simulink model "stormAD_Architecture"  (R2024a)
settings: Solver=FixedStepDiscrete  StartTime=0.0  StopTime=10.0  RelTol=1e-3
model workspace (MAT data in the model file):
  bstInterface : Simulink.Bus (value not decoded)
undefined symbols (not defined in the file): orig, RepoFilePath, UI, VisualizeDataset
(part 3 of 3)

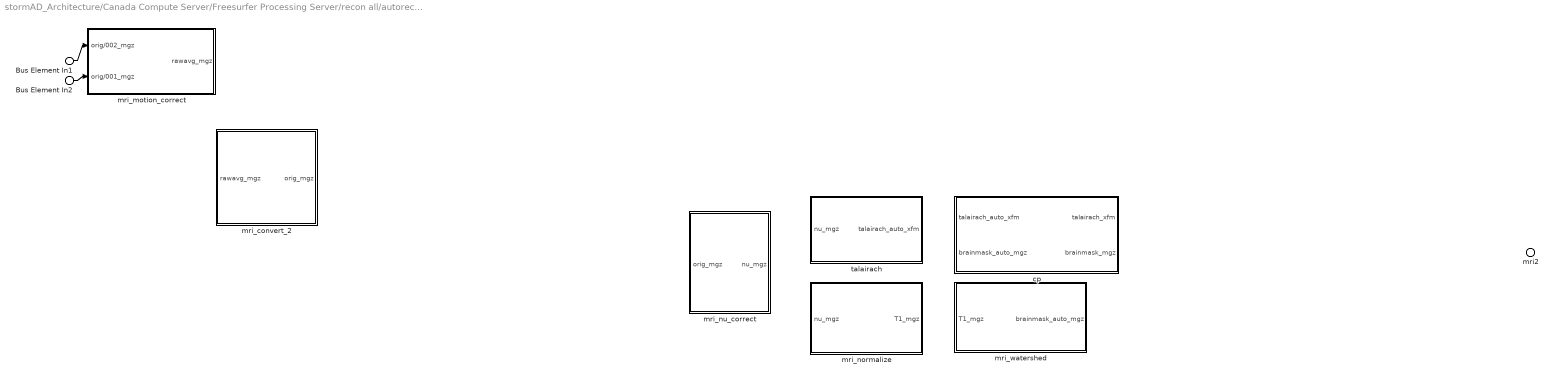
== system stormAD_Architecture/Canada Compute Server/Freesurfer Processing Server/recon all/autorecon1 ==
  Bus Element In2 : Inport  PortName=orig/001_mgz
  Bus Element In1 : Inport  Port=2  PortName=orig/002_mgz
  cp : Subsystem
      settings: PortSchema="{\"entries\":[{\"content\":{\"headerSize\":26,\"margin\":15,\"minimumSpacing\":25,\"sides\":[{\"content\":{\"connectorIds\":[\"In1\",\"In2\"]},\"type\":\"ConnectorPlacement.EquallySpacedRectSide\",\"uuid\":\"d99db108-8c8a-4010-81b2-f142fbf318f5\"},{\"content\":{\"connectorIds\":[\"Out1\",\"Out2\"],\"side\":\"RIGHT\"},\"type\":\"ConnectorPlacement.EquallySpacedRectSide\",\"uuid\":\"9190d96c-22e3-4cc9-a507-8f094dc67743\"},{\"content\":{\"side\":\"TOP\"},\"type\":\"ConnectorPlacement.EquallySpacedRectSide\",\"uuid\":\"08b46875-eac1-4edb-b2eb-5598dd517a75\"}]},\"type\":\"ConnectorPlacement.EquallySpacedConnector\",\"uuid\":\"c8d2d02b-cf5a-431f-8876-22d36c8a9b33\"}],\"packageUris\":[\"http://schema.mathworks.com/mf0/Connector/R2020b\"],\"version\":\"1.0\"}"
  mri_convert_2 : Subsystem
      settings: PortSchema="{\"entries\":[{\"content\":{\"headerSize\":26,\"margin\":15,\"minimumSpacing\":25,\"sides\":[{\"content\":{\"connectorIds\":[\"In1\"]},\"type\":\"ConnectorPlacement.EquallySpacedRectSide\",\"uuid\":\"d99db108-8c8a-4010-81b2-f142fbf318f5\"},{\"content\":{\"connectorIds\":[\"Out1\"],\"side\":\"RIGHT\"},\"type\":\"ConnectorPlacement.EquallySpacedRectSide\",\"uuid\":\"9190d96c-22e3-4cc9-a507-8f094dc67743\"},{\"content\":{\"side\":\"TOP\"},\"type\":\"ConnectorPlacement.EquallySpacedRectSide\",\"uuid\":\"08b46875-eac1-4edb-b2eb-5598dd517a75\"}]},\"type\":\"ConnectorPlacement.EquallySpacedConnector\",\"uuid\":\"c8d2d02b-cf5a-431f-8876-22d36c8a9b33\"}],\"packageUris\":[\"http://schema.mathworks.com/mf0/Connector/R2020b\"],\"version\":\"1.0\"}"
  mri_motion_correct : Subsystem
      settings: PortSchema="{\"entries\":[{\"content\":{\"headerSize\":26,\"margin\":15,\"minimumSpacing\":25,\"sides\":[{\"content\":{\"connectorIds\":[\"In1\",\"In2\"]},\"type\":\"ConnectorPlacement.EquallySpacedRectSide\",\"uuid\":\"d99db108-8c8a-4010-81b2-f142fbf318f5\"},{\"content\":{\"connectorIds\":[\"Out1\"],\"side\":\"RIGHT\"},\"type\":\"ConnectorPlacement.EquallySpacedRectSide\",\"uuid\":\"9190d96c-22e3-4cc9-a507-8f094dc67743\"},{\"content\":{\"side\":\"TOP\"},\"type\":\"ConnectorPlacement.EquallySpacedRectSide\",\"uuid\":\"08b46875-eac1-4edb-b2eb-5598dd517a75\"}]},\"type\":\"ConnectorPlacement.EquallySpacedConnector\",\"uuid\":\"c8d2d02b-cf5a-431f-8876-22d36c8a9b33\"}],\"packageUris\":[\"http://schema.mathworks.com/mf0/Connector/R2020b\"],\"version\":\"1.0\"}"
  mri_normalize : Subsystem
      settings: PortSchema="{\"entries\":[{\"content\":{\"headerSize\":26,\"margin\":15,\"minimumSpacing\":25,\"sides\":[{\"content\":{\"connectorIds\":[\"In1\"]},\"type\":\"ConnectorPlacement.EquallySpacedRectSide\",\"uuid\":\"d99db108-8c8a-4010-81b2-f142fbf318f5\"},{\"content\":{\"connectorIds\":[\"Out1\"],\"side\":\"RIGHT\"},\"type\":\"ConnectorPlacement.EquallySpacedRectSide\",\"uuid\":\"9190d96c-22e3-4cc9-a507-8f094dc67743\"},{\"content\":{\"side\":\"TOP\"},\"type\":\"ConnectorPlacement.EquallySpacedRectSide\",\"uuid\":\"08b46875-eac1-4edb-b2eb-5598dd517a75\"}]},\"type\":\"ConnectorPlacement.EquallySpacedConnector\",\"uuid\":\"c8d2d02b-cf5a-431f-8876-22d36c8a9b33\"}],\"packageUris\":[\"http://schema.mathworks.com/mf0/Connector/R2020b\"],\"version\":\"1.0\"}"
  mri_nu_correct : Subsystem
      settings: PortSchema="{\"entries\":[{\"content\":{\"headerSize\":26,\"margin\":15,\"minimumSpacing\":25,\"sides\":[{\"content\":{\"connectorIds\":[\"In1\"]},\"type\":\"ConnectorPlacement.EquallySpacedRectSide\",\"uuid\":\"d99db108-8c8a-4010-81b2-f142fbf318f5\"},{\"content\":{\"connectorIds\":[\"Out1\"],\"side\":\"RIGHT\"},\"type\":\"ConnectorPlacement.EquallySpacedRectSide\",\"uuid\":\"9190d96c-22e3-4cc9-a507-8f094dc67743\"},{\"content\":{\"side\":\"TOP\"},\"type\":\"ConnectorPlacement.EquallySpacedRectSide\",\"uuid\":\"08b46875-eac1-4edb-b2eb-5598dd517a75\"}]},\"type\":\"ConnectorPlacement.EquallySpacedConnector\",\"uuid\":\"c8d2d02b-cf5a-431f-8876-22d36c8a9b33\"}],\"packageUris\":[\"http://schema.mathworks.com/mf0/Connector/R2020b\"],\"version\":\"1.0\"}"
  mri_watershed : Subsystem
      settings: PortSchema="{\"entries\":[{\"content\":{\"headerSize\":26,\"margin\":15,\"minimumSpacing\":25,\"sides\":[{\"content\":{\"connectorIds\":[\"In1\"]},\"type\":\"ConnectorPlacement.EquallySpacedRectSide\",\"uuid\":\"d99db108-8c8a-4010-81b2-f142fbf318f5\"},{\"content\":{\"connectorIds\":[\"Out1\"],\"side\":\"RIGHT\"},\"type\":\"ConnectorPlacement.EquallySpacedRectSide\",\"uuid\":\"9190d96c-22e3-4cc9-a507-8f094dc67743\"},{\"content\":{\"side\":\"TOP\"},\"type\":\"ConnectorPlacement.EquallySpacedRectSide\",\"uuid\":\"08b46875-eac1-4edb-b2eb-5598dd517a75\"}]},\"type\":\"ConnectorPlacement.EquallySpacedConnector\",\"uuid\":\"c8d2d02b-cf5a-431f-8876-22d36c8a9b33\"}],\"packageUris\":[\"http://schema.mathworks.com/mf0/Connector/R2020b\"],\"version\":\"1.0\"}"
  talairach : Subsystem
      settings: PortSchema="{\"entries\":[{\"content\":{\"headerSize\":26,\"margin\":15,\"minimumSpacing\":25,\"sides\":[{\"content\":{\"connectorIds\":[\"In1\"]},\"type\":\"ConnectorPlacement.EquallySpacedRectSide\",\"uuid\":\"d99db108-8c8a-4010-81b2-f142fbf318f5\"},{\"content\":{\"connectorIds\":[\"Out1\"],\"side\":\"RIGHT\"},\"type\":\"ConnectorPlacement.EquallySpacedRectSide\",\"uuid\":\"9190d96c-22e3-4cc9-a507-8f094dc67743\"},{\"content\":{\"side\":\"TOP\"},\"type\":\"ConnectorPlacement.EquallySpacedRectSide\",\"uuid\":\"08b46875-eac1-4edb-b2eb-5598dd517a75\"}]},\"type\":\"ConnectorPlacement.EquallySpacedConnector\",\"uuid\":\"c8d2d02b-cf5a-431f-8876-22d36c8a9b33\"}],\"packageUris\":[\"http://schema.mathworks.com/mf0/Connector/R2020b\"],\"version\":\"1.0\"}"
  mri2 : Outport  PortName=mri1
  wires:
  Bus Element In1/1 -> mri_motion_correct/1(orig/002_mgz)
  Bus Element In2/1 -> mri_motion_correct/2(orig/001_mgz)

== system stormAD_Architecture/Canada Compute Server/Freesurfer Processing Server/recon all/autorecon2 ==
  Bus Element In1 : Inport  PortName=InBus

== system stormAD_Architecture/Canada Compute Server/Freesurfer Processing Server/recon all/autorecon3 ==

== system stormAD_Architecture/Canada Compute Server/Freesurfer Processing Server/recon all/labelDirectory ==
  Bus Element Out1 : Outport  PortName=label

== system stormAD_Architecture/Canada Compute Server/Freesurfer Processing Server/recon all/mriDirectory ==
  Bus Element Out1 : Outport  PortName=mri

== system stormAD_Architecture/Canada Compute Server/Freesurfer Processing Server/recon all/mri_convert ==
  Bus Element In2 : Inport  AllowServiceAccess=on  PortName=Data
  Bus Element Out2 : Outport  PortName=orig/002_mgz
  Bus Element Out1 : Outport  Port=2  PortName=orig/001_mgz

== system stormAD_Architecture/Canada Compute Server/Freesurfer Processing Server/recon all/scriptsDirectory ==
  Bus Element Out1 : Outport  PortName=scripts

== system stormAD_Architecture/Canada Compute Server/Freesurfer Processing Server/recon all/statsDirectory ==
  Bus Element Out1 : Outport  PortName=stats

== system stormAD_Architecture/Canada Compute Server/Freesurfer Processing Server/recon all/subjectDirectory ==
  Bus Element In7 : Inport  PortName=tmp
  Bus Element In6 : Inport  Port=2  PortName=mri
  Bus Element In2 : Inport  Port=3  PortName=scripts
  Bus Element In3 : Inport  Port=4  PortName=surf
  Bus Element In1 : Inport  Port=5  PortName=stats
  Bus Element In4 : Inport  Port=6  PortName=trash
  Bus Element In5 : Inport  Port=7  PortName=label
  Bus Element Out1 : Outport  PortName=subject

== system stormAD_Architecture/Canada Compute Server/Freesurfer Processing Server/recon all/surfDirectory ==
  Bus Element Out1 : Outport  PortName=surf

== system stormAD_Architecture/Canada Compute Server/Freesurfer Processing Server/recon all/tmpDirectory ==
  Bus Element Out1 : Outport  PortName=tmp

== system stormAD_Architecture/Canada Compute Server/Freesurfer Processing Server/recon all/trashDirectory ==
  Bus Element Out1 : Outport  PortName=trash

== system stormAD_Architecture/Data Management/Dataset ORM/RepoReader/cleanRepo ==
  Bus Element In1 : Inport  PortName=InBus
  Bus Element Out1 : Outport  PortName=OutBus

== system stormAD_Architecture/Data Management/Dataset ORM/RepoReader/listDirectories ==
  Bus Element In1 : Inport  PortName=UI-RepoFilePath
  Bus Element Out1 : Outport  PortName=OutBus

== system stormAD_Architecture/Data Management/Dataset ORM/RepoReader/map ==
  Bus Element In1 : Inport  PortName=InBus
  Bus Element Out1 : Outport  PortName=RepoMap
  Bus Element Out2 : Outport  Port=2  PortName=syncrhonize_DB

== system stormAD_Architecture/StormAD Core/PET/regionStat/maskSelector ==
  Bus Element In2 : Inport  PortName=maskUI
  Bus Element In1 : Inport  Port=2  PortName=anat4pet
  Bus Element Out1 : Outport  PortName=mask

== system stormAD_Architecture/StormAD Core/PET/regionStat/smoothedPET ==
  Bus Element In1 : Inport  PortName=mask

== system stormAD_Architecture/Canada Compute Server/Freesurfer Processing Server/recon all/autorecon1/cp ==
  Bus Element In1 : Inport  PortName=talairach_auto_xfm
  Bus Element In2 : Inport  Port=2  PortName=brainmask_auto_mgz
  Bus Element Out1 : Outport  PortName=talairach_xfm
  Bus Element Out2 : Outport  Port=2  PortName=brainmask_mgz

== system stormAD_Architecture/Canada Compute Server/Freesurfer Processing Server/recon all/autorecon1/mri_convert_2 ==
  Bus Element In1 : Inport  PortName=rawavg_mgz
  Bus Element Out1 : Outport  PortName=orig_mgz

== system stormAD_Architecture/Canada Compute Server/Freesurfer Processing Server/recon all/autorecon1/mri_motion_correct ==
  Bus Element In1 : Inport  PortName=orig/002_mgz
  Bus Element In2 : Inport  Port=2  PortName=orig/001_mgz
  Bus Element Out1 : Outport  PortName=rawavg_mgz

== system stormAD_Architecture/Canada Compute Server/Freesurfer Processing Server/recon all/autorecon1/mri_normalize ==
  Bus Element In1 : Inport  PortName=nu_mgz
  Bus Element Out1 : Outport  PortName=T1_mgz

== system stormAD_Architecture/Canada Compute Server/Freesurfer Processing Server/recon all/autorecon1/mri_nu_correct ==
  Bus Element In1 : Inport  PortName=orig_mgz
  Bus Element Out1 : Outport  PortName=nu_mgz

== system stormAD_Architecture/Canada Compute Server/Freesurfer Processing Server/recon all/autorecon1/mri_watershed ==
  Bus Element In1 : Inport  PortName=T1_mgz
  Bus Element Out1 : Outport  PortName=brainmask_auto_mgz

== system stormAD_Architecture/Canada Compute Server/Freesurfer Processing Server/recon all/autorecon1/talairach ==
  Bus Element In1 : Inport  PortName=nu_mgz
  Bus Element Out1 : Outport  PortName=talairach_auto_xfm
